simulink model "case 3"  (R2018a)
settings: Solver=VariableStepAuto  StartTime=0.0  StopTime=5  RelTol=1e-3
values from neighbouring files (symbols this model uses):
  cdcc = 0.00022    [matlab.mat]
  cf = 8e-05    [matlab.mat]
  iodmax = 12    [matlab.mat]
  iqdmax = -7.2    [matlab.mat]
  kiid = 0.5    [matlab.mat]
  kiiq = -5    [matlab.mat]
  kpid = 0.4    [matlab.mat]
  kpiq = -4    [matlab.mat]
  lf = 0.0075    [matlab.mat]
  ll = 1e-06    [matlab.mat]
  md = 0.001    [matlab.mat]
  nq = 0.002    [matlab.mat]
  p0 = 240    [matlab.mat]
  q0 = 60    [matlab.mat]
  rf = 0.0015    [matlab.mat]
  rl = 0.001    [matlab.mat]
  vdc = 200    [matlab.mat]
  wc = 0.000125663706144    [matlab.mat]
undefined symbols (not defined in the file or in its folder): DiscIntNeverNeededParam, gcbh, sps, sps_rtmsupport
libraries: neural x30, powerlib_meascontrol x27, powerlib x17, spsVIMeasurementModel x6, simulink x4, spsMeanValueModel x2
(part 1 of 2)
settings Model: Creator=Febin  LastModifiedBy=febin

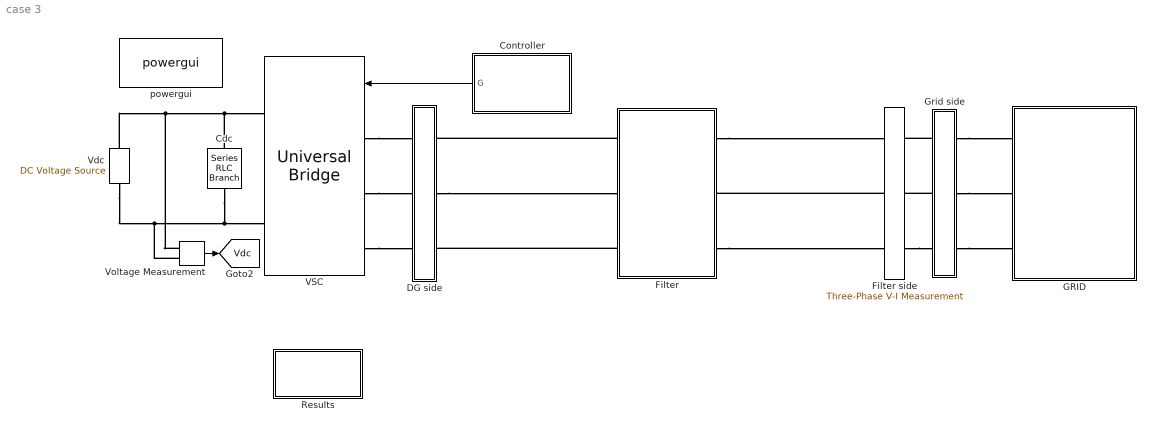
== system case 3 ==
  Cdc : powerlib/Elements/Series RLC Branch  LConnTagsString=__new0  RConnTagsString=__new0  BranchType=RC  Resistance=0.0001  Inductance=1e-3  SetiL0=off  InitialCurrent=0  Capacitance=cdcc  Setx0=off  InitialVoltage=0  Measurements=None
  Controller : Subsystem
  DG side : Subsystem  DialogController=POWERSYS.PowerSysDialog  LoadFcn=|  StartFcn=sps_rtmsupport('StartFcn',gcbh);  StopFcn=sps_rtmsupport('StopFcn',gcbh);  mask(Three-Phase VI Measurement){VoltageMeasurement=phase-to-ground, SetLabelV=on, LabelV=vabc, Vpu=off, VpuLL=off, CurrentMeasurement=yes, SetLabelI=on, LabelI=iabc, Ipu=off, Pbase=100e6, Vbase=500e3, OutputType=Complex, PhasorSimulation=off, PSBequivalent=0}
      | if ~strcmp(get_param(bdroot,'BlockDiagramType'),'library')
      |     set_param([gcb,'/Model'],'LinkStatus','restore');
      | end
      | sps_rtmsupport('LoadFcn',gcbh);
      mask prompts: VoltageMeasurement "Voltage measurement"; SetLabelV "Use a label"; LabelV "Signal label  (use a From block to collect this signal)"; Vpu "Voltages in pu,  based on peak value of nominal phase-to-ground voltage"; VpuLL "Voltages in pu,  based on peak value of nominal phase-to-phase  voltage"; CurrentMeasurement "Current measurement"; SetLabelI "Use a label"; LabelI "Signal label  (use a From block to collect this signal)"; Ipu "Currents in pu"; Pbase "Base power ( VA 3 phase)"; Vbase "Nominal voltage used for pu measurement (Vrms phase-phase) :"; OutputType "Output signals in:"; PhasorSimulation "Phasor simulation (internal use)"; PSBequivalent "Equivalent circuit (internal use)"
      mask help:
      | Ideal three-phase voltage and current measurements.
      |
      | The block can output the voltages and currents in per unit values or in volts and amperes.
      mask init:
      | block = gcb;
      | Kv=1;
      | Ki=1;
      | [Kv,Ki] = powericon('ThreePhaseVIMeasurementParam',block,Vpu,VpuLL,Ipu,Vbase,Pbase,PhasorSimulation,OutputType);
      | powericon('ThreePhaseVIMeasurementCback',block);
      | power_initmask();
      settings: CopyFcn=sps_rtmsupport('CopyFcn',gcbh); powericon('ThreePhaseVIMeasurementCopy',gcb)  DeleteFcn=sps_rtmsupport('DeleteFcn',gcbh);  UndoDeleteFcn=sps_rtmsupport('UndoDeleteFcn',gcbh);  ModelCloseFcn=sps_rtmsupport('ModelCloseFcn',gcbh);  PostSaveFcn=sps_rtmsupport('PostSaveFcn',gcbh);  NameChangeFcn=sps_rtmsupport('NameChangeFcn',gcbh);  PreCopyFcn=sps_rtmsupport('PreCopyFcn',gcbh);  OpenFcn=sps_rtmsupport('OpenFcn',gcbh, [1 2 4 5 6 7 9 -12 13]);  CloseFcn=sps_rtmsupport('CloseFcn',gcbh);  PreDeleteFcn=sps_rtmsupport('PreDeleteFcn',gcbh);
      settings: PreSaveFcn=|
      | sps_rtmsupport('PreSaveFcn',gcbh);
      | if ~strcmp(get_param(bdroot(gcbh),'BlockDiagramType'),'library')
      |     set_param(gcb,'LinkStatus','restore')
      | end
      mask Help: helpview(psbhelp)
      mask TypeOptions VoltageMeasurement: no | phase-to-ground | phase-to-phase
      mask Callback VoltageMeasurement: powericon('ThreePhaseVIMeasurementCback',gcb,'Vselector');
      mask Callback SetLabelV: powericon('ThreePhaseVIMeasurementCback',gcb,'');
      mask Callback Vpu: powericon('ThreePhaseVIMeasurementCback',gcb,'Vpu');
      mask Callback VpuLL: powericon('ThreePhaseVIMeasurementCback',gcb,'VpuLL');
      mask TypeOptions CurrentMeasurement: no | yes
      mask Callback CurrentMeasurement: powericon('ThreePhaseVIMeasurementCback',gcb,'');
      mask Callback SetLabelI: powericon('ThreePhaseVIMeasurementCback',gcb,'');
      mask Callback LabelI: powericon('ThreePhaseVIMeasurementCback',gcb,'');
      mask Callback Ipu: powericon('ThreePhaseVIMeasurementCback',gcb,'');
      mask TypeOptions OutputType: Complex | Real-Imag | Magnitude-Angle | Magnitude
  Filter : Subsystem
  Filter side : powerlib/Measurements/Three-Phase V-I Measurement  VoltageMeasurement=phase-to-ground  SetLabelV=on  LabelV=v0abc  Vpu=off  VpuLL=off  CurrentMeasurement=yes  SetLabelI=on  LabelI=i0abc  Ipu=off  Pbase=100e6  Vbase=500e3  OutputType=Complex  PhasorSimulation=off  PSBequivalent=0
  GRID : Subsystem
  Grid side : Subsystem  DialogController=POWERSYS.PowerSysDialog  LoadFcn=|  StartFcn=sps_rtmsupport('StartFcn',gcbh);  StopFcn=sps_rtmsupport('StopFcn',gcbh);  mask(Three-Phase VI Measurement){VoltageMeasurement=phase-to-ground, SetLabelV=on, LabelV=vgabc, Vpu=off, VpuLL=off, CurrentMeasurement=yes, SetLabelI=on, LabelI=igabc, Ipu=off, Pbase=100e6, Vbase=500e3, OutputType=Complex, PhasorSimulation=off, PSBequivalent=0}
      | if ~strcmp(get_param(bdroot,'BlockDiagramType'),'library')
      |     set_param([gcb,'/Model'],'LinkStatus','restore');
      | end
      | sps_rtmsupport('LoadFcn',gcbh);
      mask prompts: VoltageMeasurement "Voltage measurement"; SetLabelV "Use a label"; LabelV "Signal label  (use a From block to collect this signal)"; Vpu "Voltages in pu,  based on peak value of nominal phase-to-ground voltage"; VpuLL "Voltages in pu,  based on peak value of nominal phase-to-phase  voltage"; CurrentMeasurement "Current measurement"; SetLabelI "Use a label"; LabelI "Signal label  (use a From block to collect this signal)"; Ipu "Currents in pu"; Pbase "Base power ( VA 3 phase)"; Vbase "Nominal voltage used for pu measurement (Vrms phase-phase) :"; OutputType "Output signals in:"; PhasorSimulation "Phasor simulation (internal use)"; PSBequivalent "Equivalent circuit (internal use)"
      mask help:
      | Ideal three-phase voltage and current measurements.
      |
      | The block can output the voltages and currents in per unit values or in volts and amperes.
      mask init: same as case 3/DG side
      settings: CopyFcn=sps_rtmsupport('CopyFcn',gcbh); powericon('ThreePhaseVIMeasurementCopy',gcb)  DeleteFcn=sps_rtmsupport('DeleteFcn',gcbh);  UndoDeleteFcn=sps_rtmsupport('UndoDeleteFcn',gcbh);  ModelCloseFcn=sps_rtmsupport('ModelCloseFcn',gcbh);  PostSaveFcn=sps_rtmsupport('PostSaveFcn',gcbh);  NameChangeFcn=sps_rtmsupport('NameChangeFcn',gcbh);  PreCopyFcn=sps_rtmsupport('PreCopyFcn',gcbh);  OpenFcn=sps_rtmsupport('OpenFcn',gcbh, [1 2 4 5 6 7 9 -12 13]);  CloseFcn=sps_rtmsupport('CloseFcn',gcbh);  PreDeleteFcn=sps_rtmsupport('PreDeleteFcn',gcbh);
      settings: PreSaveFcn=|
      | sps_rtmsupport('PreSaveFcn',gcbh);
      | if ~strcmp(get_param(bdroot(gcbh),'BlockDiagramType'),'library')
      |     set_param(gcb,'LinkStatus','restore')
      | end
      mask Help: helpview(psbhelp)
      mask TypeOptions VoltageMeasurement: no | phase-to-ground | phase-to-phase
      mask Callback VoltageMeasurement: powericon('ThreePhaseVIMeasurementCback',gcb,'Vselector');
      mask Callback SetLabelV: powericon('ThreePhaseVIMeasurementCback',gcb,'');
      mask Callback Vpu: powericon('ThreePhaseVIMeasurementCback',gcb,'Vpu');
      mask Callback VpuLL: powericon('ThreePhaseVIMeasurementCback',gcb,'VpuLL');
      mask TypeOptions CurrentMeasurement: no | yes
      mask Callback CurrentMeasurement: powericon('ThreePhaseVIMeasurementCback',gcb,'');
      mask Callback SetLabelI: powericon('ThreePhaseVIMeasurementCback',gcb,'');
      mask Callback LabelI: powericon('ThreePhaseVIMeasurementCback',gcb,'');
      mask Callback Ipu: powericon('ThreePhaseVIMeasurementCback',gcb,'');
      mask TypeOptions OutputType: Complex | Real-Imag | Magnitude-Angle | Magnitude
  Results : Subsystem
  VSC : powerlib/Power Electronics/Universal Bridge  Arms=3  SnubberResistance=1e5  SnubberCapacitance=inf  Device=IGBT / Diodes  Ron=1e-3  Lon=0  ForwardVoltages="[  0  0  ]"  ForwardVoltage=0  GTOparameters=[ 10e-6 , 20e-6 ]  IGBTparameters=[ 1e-6 , 2e-6 ]  Measurements=None  Measurements_2=None  converterType=Rectifier
  Vdc : powerlib/Electrical Sources/DC Voltage Source  Amplitude=vdc  Measurements=None
  Voltage Measurement : powerlib/Measurements/Voltage Measurement  PhasorSimulation=off  OutputType=Complex  PSBequivalent=0
  powergui : powerlib/powergui  Priority=1  SimulationMode=Discrete  SampleTime=50e-6  frequency=60  Iterations=50  frequencyindice=0  Pbase=100e6  ErrMax=1e-4  UnitsV=kV  UnitsW=MW  buscounter=0  FunctionMessages=off  echomessages=off  EnableUseOfTLC=off  CurrentSourceSwitches=off  DisableSnubberDevices=off  DisableRonSwitches=off  DisableVfSwitches=off  DisplayEquations=off  SolverType=Tustin/Backward Euler (TBE)  Interpol=off  ExternalGateDelay=off  methode=off  Ts=100  x0status=blocks  SPID=off  SwTol=0  HookPort=off  RestoreLinks=warning  ResistiveCurrentMeasurement=off  Frange=[0:2:500]  Ylog=off  Xlog=on  ShowGrid=off  save=off  variable=ZData  structure=0  ZoomFFT=on  StartTime=0.0  cycles=1  DisplayStyle=1  fundamental=60  FreqAxis=off  MaxFrequency=1000  frequencyindicesteady=1  RmsSteady=1  display=off
  tag scope: Vdc=global
  wires:
  Controller/1(G) -> VSC/1
  Voltage Measurement/1 -> [Vdc]
  connections:
  Vdc/RConn1 -- Voltage Measurement/LConn1 -- Cdc/LConn1 -- VSC/RConn1
  Vdc/LConn1 -- Voltage Measurement/LConn2 -- Cdc/RConn1 -- VSC/RConn2
  VSC/LConn3 -- DG side/LConn3
  VSC/LConn2 -- DG side/LConn2
  VSC/LConn1 -- DG side/LConn1
  Grid side/RConn1 -- Filter side/LConn1
  Grid side/RConn2 -- Filter side/LConn2
  Filter side/LConn3 -- Grid side/RConn3
  Grid side/LConn1 -- GRID/RConn1
  Grid side/LConn2 -- GRID/RConn2
  Grid side/LConn3 -- GRID/RConn3
  Filter/LConn1 -- DG side/RConn1
  Filter/RConn1 -- Filter side/RConn1
  DG side/RConn2 -- Filter/LConn2
  Filter side/RConn2 -- Filter/RConn2
  Filter/LConn3 -- DG side/RConn3
  Filter/RConn3 -- Filter side/RConn3

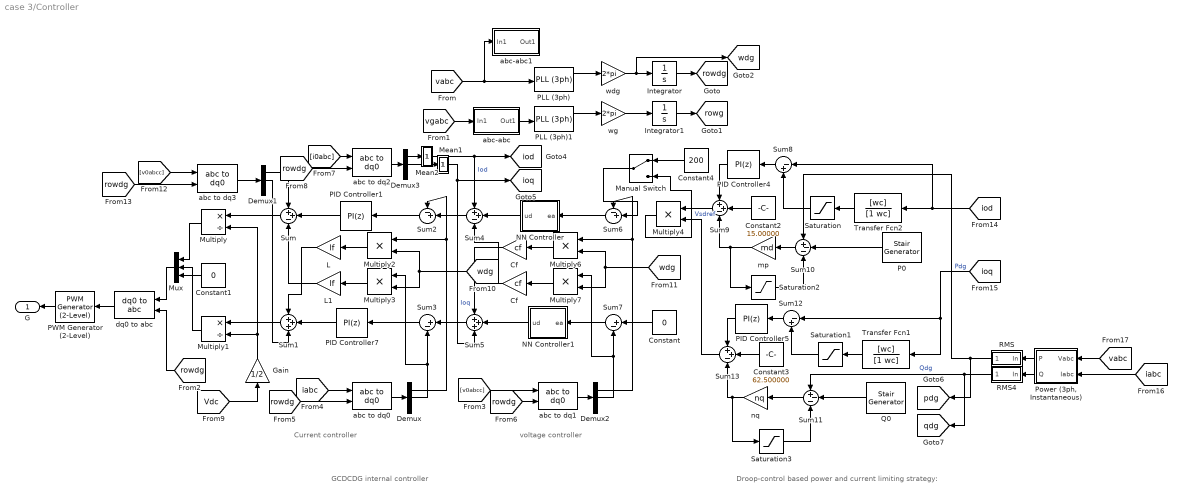
== system case 3/Controller ==
  note: voltage controller
  note: Current controller
  note: GCDCDG internal controller
  note: Droop-control based power and current limiting strategy:
  Cf : Gain  Gain=cf
  "Cf " : Gain  Gain=cf
  Constant : Constant  Value=0
  Constant1 : Constant  Value=0
  Constant2 : Constant  Value=15.00000
  Constant3 : Constant  Value=62.500000
  Constant4 : Constant  Value=200
  Demux{,1..3} (4 alike) : Demux  Outputs=3
  Gain : Gain  Gain=1/2
  Integrator : Integrator
  Integrator1 : Integrator
  L : Gain  Gain=lf
  L1 : Gain  Gain=lf
  Manual Switch : ManualSwitch
  Mean1 : Subsystem  DialogController=POWERSYS.PowerSysDialog  LoadFcn=sps_rtmsupport('LoadFcn', gcbh);  StartFcn=sps_rtmsupport('StartFcn', gcbh);  StopFcn=sps_rtmsupport('StopFcn', gcbh);  mask(Mean){Freq=50, Vinit=0, Ts=50e-6}
      mask prompts: Freq "Fundamental frequency (Hz):"; Vinit "Initial input (DC component):"; Ts "Sample time:"
      mask help: Compute the mean value of the input signal over a running window of one cycle of the specified fundamental frequency. For the first cycle of simulation, the output is held constant to the specified initial input value.
      mask init:
      | block=gcb;
      | [WantBlockChoice,Ts,sps] = powericon('MeanInit',block,Freq,Vinit,Ts);
      | powericon('SetInternalModels','set',block,WantBlockChoice);
      settings: CopyFcn=sps_rtmsupport('CopyFcn', gcbh);  DeleteFcn=sps_rtmsupport('DeleteFcn', gcbh);  UndoDeleteFcn=sps_rtmsupport('UndoDeleteFcn', gcbh);  ModelCloseFcn=sps_rtmsupport('ModelCloseFcn', gcbh);  PreSaveFcn=sps_rtmsupport('PreSaveFcn', gcbh);  PostSaveFcn=sps_rtmsupport('PostSaveFcn', gcbh);  NameChangeFcn=sps_rtmsupport('NameChangeFcn', gcbh);  PreCopyFcn=sps_rtmsupport('PreCopyFcn', gcbh);  OpenFcn=sps_rtmsupport('OpenFcn', gcbh, []);  CloseFcn=sps_rtmsupport('CloseFcn', gcbh);  PreDeleteFcn=sps_rtmsupport('PreDeleteFcn', gcbh);
      mask Help: helpview(psbhelp);
      mask Display:
      | plot(0,0, 1,1)
      | plot([0.8 1], [0.75 0.75])
      | plot([0.85 .95], [0.35 0.65],[0.85 .95], [0.65 0.35])
  Mean2 : Subsystem  DialogController=POWERSYS.PowerSysDialog  LoadFcn=sps_rtmsupport('LoadFcn', gcbh);  StartFcn=sps_rtmsupport('StartFcn', gcbh);  StopFcn=sps_rtmsupport('StopFcn', gcbh);  mask(Mean){Freq=50, Vinit=0, Ts=50e-6}
      mask prompts: Freq "Fundamental frequency (Hz):"; Vinit "Initial input (DC component):"; Ts "Sample time:"
      mask help: Compute the mean value of the input signal over a running window of one cycle of the specified fundamental frequency. For the first cycle of simulation, the output is held constant to the specified initial input value.
      mask init:
      | block=gcb;
      | [WantBlockChoice,Ts,sps] = powericon('MeanInit',block,Freq,Vinit,Ts);
      | powericon('SetInternalModels','set',block,WantBlockChoice);
      settings: CopyFcn=sps_rtmsupport('CopyFcn', gcbh);  DeleteFcn=sps_rtmsupport('DeleteFcn', gcbh);  UndoDeleteFcn=sps_rtmsupport('UndoDeleteFcn', gcbh);  ModelCloseFcn=sps_rtmsupport('ModelCloseFcn', gcbh);  PreSaveFcn=sps_rtmsupport('PreSaveFcn', gcbh);  PostSaveFcn=sps_rtmsupport('PostSaveFcn', gcbh);  NameChangeFcn=sps_rtmsupport('NameChangeFcn', gcbh);  PreCopyFcn=sps_rtmsupport('PreCopyFcn', gcbh);  OpenFcn=sps_rtmsupport('OpenFcn', gcbh, []);  CloseFcn=sps_rtmsupport('CloseFcn', gcbh);  PreDeleteFcn=sps_rtmsupport('PreDeleteFcn', gcbh);
      mask Help: helpview(psbhelp);
      mask Display:
      | plot(0,0, 1,1)
      | plot([0.8 1], [0.75 0.75])
      | plot([0.85 .95], [0.35 0.65],[0.85 .95], [0.65 0.35])
  Multiply : Product  Inputs=*/
  Multiply1 : Product  Inputs=*/
  Multiply{2..4,6..7} (5 alike) : Product
  Mux : Mux  Inputs=3
  NN Controller : Subsystem
  NN Controller1 : Subsystem
  P0 : powerlib_meascontrol/Pulse & Signal Generators/Stair Generator  t=[0 2 5]  e=[1 1 1]*p0  Ts=50e-6
      settings: SourceProductName=Simscape Power Systems
  PID Controller1 : simulink/Continuous/PID Controller  Controller=PI  TimeDomain=Discrete-time  SampleTime=-1  IntegratorMethod=Forward Euler  FilterMethod=Forward Euler  Form=Parallel  UseFilter=on  ControllerParametersSource=internal  P=0.2  I=0.01  D=0  N=100  InitialConditionSource=internal  InitialConditionForIntegrator=0  InitialConditionForFilter=0  ExternalReset=none  LimitOutput=off  UpperSaturationLimit=1  LowerSaturationLimit=-1  LinearizeAsGain=on  AntiWindupMode=none  Kb=1  TrackingMode=off  Kt=1  PParamMin=[]  PParamMax=[]  IParamMin=[]  IParamMax=[]  DParamMin=[]  DParamMax=[]  NParamMin=[]  NParamMax=[]  KbParamMin=[]  KbParamMax=[]  KtParamMin=[]  KtParamMax=[]  POutMin=[]  POutMax=[]  IOutMin=[]  IOutMax=[]  DOutMin=[]  DOutMax=[]  NOutMin=[]  NOutMax=[]  KbOutMin=[]  KbOutMax=[]  KtOutMin=[]  KtOutMax=[]  IntegratorOutMin=[]  IntegratorOutMax=[]  FilterOutMin=[]  FilterOutMax=[]  SumOutMin=[]  SumOutMax=[]  SumI1OutMin=[]  SumI1OutMax=[]  SumI2OutMin=[]  SumI2OutMax=[]  SumI3OutMin=[]  SumI3OutMax=[]  SumDOutMin=[]  SumDOutMax=[]  SaturationOutMin=[]  SaturationOutMax=[]  IntegratorContinuousStateAttributes=''  IntegratorStateMustResolveToSignalObject=off  IntegratorRTWStateStorageClass=Auto  FilterContinuousStateAttributes=''  FilterStateMustResolveToSignalObject=off  FilterRTWStateStorageClass=Auto  DifferentiatorICPrevScaledInput=0  DifferentiatorOutMin=[]  DifferentiatorOutMax=[]  FilterDiffOutCoefMin=[]  FilterDiffOutCoefMax=[]  SumDenOutMin=[]  SumDenOutMax=[]  SumNumOutMin=[]  SumNumOutMax=[]  ReciprocalOutMin=[]  ReciprocalOutMax=[]  DivideOutMin=[]  DivideOutMax=[]  TunerSelectOption=Transfer Function Based (PID Tuner App)
  PID Controller4 : simulink/Continuous/PID Controller  Controller=PI  TimeDomain=Discrete-time  SampleTime=-1  IntegratorMethod=Forward Euler  FilterMethod=Forward Euler  Form=Parallel  UseFilter=on  ControllerParametersSource=internal  P=kpid  I=kpiq  D=0  N=100  InitialConditionSource=internal  InitialConditionForIntegrator=0  InitialConditionForFilter=0  ExternalReset=none  LimitOutput=off  UpperSaturationLimit=inf  LowerSaturationLimit=-inf  LinearizeAsGain=on  AntiWindupMode=none  Kb=1  TrackingMode=off  Kt=1  PParamMin=[]  PParamMax=[]  IParamMin=[]  IParamMax=[]  DParamMin=[]  DParamMax=[]  NParamMin=[]  NParamMax=[]  KbParamMin=[]  KbParamMax=[]  KtParamMin=[]  KtParamMax=[]  POutMin=[]  POutMax=[]  IOutMin=[]  IOutMax=[]  DOutMin=[]  DOutMax=[]  NOutMin=[]  NOutMax=[]  KbOutMin=[]  KbOutMax=[]  KtOutMin=[]  KtOutMax=[]  IntegratorOutMin=[]  IntegratorOutMax=[]  FilterOutMin=[]  FilterOutMax=[]  SumOutMin=[]  SumOutMax=[]  SumI1OutMin=[]  SumI1OutMax=[]  SumI2OutMin=[]  SumI2OutMax=[]  SumI3OutMin=[]  SumI3OutMax=[]  SumDOutMin=[]  SumDOutMax=[]  SaturationOutMin=[]  SaturationOutMax=[]  IntegratorContinuousStateAttributes=''  IntegratorStateMustResolveToSignalObject=off  IntegratorRTWStateStorageClass=Auto  FilterContinuousStateAttributes=''  FilterStateMustResolveToSignalObject=off  FilterRTWStateStorageClass=Auto  DifferentiatorICPrevScaledInput=0  DifferentiatorOutMin=[]  DifferentiatorOutMax=[]  FilterDiffOutCoefMin=[]  FilterDiffOutCoefMax=[]  SumDenOutMin=[]  SumDenOutMax=[]  SumNumOutMin=[]  SumNumOutMax=[]  ReciprocalOutMin=[]  ReciprocalOutMax=[]  DivideOutMin=[]  DivideOutMax=[]  TunerSelectOption=Transfer Function Based (PID Tuner App)
  PID Controller5 : simulink/Continuous/PID Controller  Controller=PI  TimeDomain=Discrete-time  SampleTime=-1  IntegratorMethod=Forward Euler  FilterMethod=Forward Euler  Form=Parallel  UseFilter=on  ControllerParametersSource=internal  P=kiid  I=kiiq  D=0  N=100  InitialConditionSource=internal  InitialConditionForIntegrator=0  InitialConditionForFilter=0  ExternalReset=none  LimitOutput=off  UpperSaturationLimit=inf  LowerSaturationLimit=-inf  LinearizeAsGain=on  AntiWindupMode=none  Kb=1  TrackingMode=off  Kt=1  PParamMin=[]  PParamMax=[]  IParamMin=[]  IParamMax=[]  DParamMin=[]  DParamMax=[]  NParamMin=[]  NParamMax=[]  KbParamMin=[]  KbParamMax=[]  KtParamMin=[]  KtParamMax=[]  POutMin=[]  POutMax=[]  IOutMin=[]  IOutMax=[]  DOutMin=[]  DOutMax=[]  NOutMin=[]  NOutMax=[]  KbOutMin=[]  KbOutMax=[]  KtOutMin=[]  KtOutMax=[]  IntegratorOutMin=[]  IntegratorOutMax=[]  FilterOutMin=[]  FilterOutMax=[]  SumOutMin=[]  SumOutMax=[]  SumI1OutMin=[]  SumI1OutMax=[]  SumI2OutMin=[]  SumI2OutMax=[]  SumI3OutMin=[]  SumI3OutMax=[]  SumDOutMin=[]  SumDOutMax=[]  SaturationOutMin=[]  SaturationOutMax=[]  IntegratorContinuousStateAttributes=''  IntegratorStateMustResolveToSignalObject=off  IntegratorRTWStateStorageClass=Auto  FilterContinuousStateAttributes=''  FilterStateMustResolveToSignalObject=off  FilterRTWStateStorageClass=Auto  DifferentiatorICPrevScaledInput=0  DifferentiatorOutMin=[]  DifferentiatorOutMax=[]  FilterDiffOutCoefMin=[]  FilterDiffOutCoefMax=[]  SumDenOutMin=[]  SumDenOutMax=[]  SumNumOutMin=[]  SumNumOutMax=[]  ReciprocalOutMin=[]  ReciprocalOutMax=[]  DivideOutMin=[]  DivideOutMax=[]  TunerSelectOption=Transfer Function Based (PID Tuner App)
  PID Controller7 : simulink/Continuous/PID Controller  Controller=PI  TimeDomain=Discrete-time  SampleTime=-1  IntegratorMethod=Forward Euler  FilterMethod=Forward Euler  Form=Parallel  UseFilter=on  ControllerParametersSource=internal  P=0.2  I=0.01  D=0  N=100  InitialConditionSource=internal  InitialConditionForIntegrator=0  InitialConditionForFilter=0  ExternalReset=none  LimitOutput=off  UpperSaturationLimit=1  LowerSaturationLimit=-1  LinearizeAsGain=on  AntiWindupMode=none  Kb=1  TrackingMode=off  Kt=1  PParamMin=[]  PParamMax=[]  IParamMin=[]  IParamMax=[]  DParamMin=[]  DParamMax=[]  NParamMin=[]  NParamMax=[]  KbParamMin=[]  KbParamMax=[]  KtParamMin=[]  KtParamMax=[]  POutMin=[]  POutMax=[]  IOutMin=[]  IOutMax=[]  DOutMin=[]  DOutMax=[]  NOutMin=[]  NOutMax=[]  KbOutMin=[]  KbOutMax=[]  KtOutMin=[]  KtOutMax=[]  IntegratorOutMin=[]  IntegratorOutMax=[]  FilterOutMin=[]  FilterOutMax=[]  SumOutMin=[]  SumOutMax=[]  SumI1OutMin=[]  SumI1OutMax=[]  SumI2OutMin=[]  SumI2OutMax=[]  SumI3OutMin=[]  SumI3OutMax=[]  SumDOutMin=[]  SumDOutMax=[]  SaturationOutMin=[]  SaturationOutMax=[]  IntegratorContinuousStateAttributes=''  IntegratorStateMustResolveToSignalObject=off  IntegratorRTWStateStorageClass=Auto  FilterContinuousStateAttributes=''  FilterStateMustResolveToSignalObject=off  FilterRTWStateStorageClass=Auto  DifferentiatorICPrevScaledInput=0  DifferentiatorOutMin=[]  DifferentiatorOutMax=[]  FilterDiffOutCoefMin=[]  FilterDiffOutCoefMax=[]  SumDenOutMin=[]  SumDenOutMax=[]  SumNumOutMin=[]  SumNumOutMax=[]  ReciprocalOutMin=[]  ReciprocalOutMax=[]  DivideOutMin=[]  DivideOutMax=[]  TunerSelectOption=Transfer Function Based (PID Tuner App)
  PLL (3ph) : powerlib_meascontrol/PLL/PLL (3ph)  Fmin=45  Par_Init=[0, 50]  ParK=[180, 3200, 1]  TcD=1e-4  MaxRateChangeFreq=12  FilterCutOffFreq=25  Ts=50e-6  AGC=on
  PLL (3ph)1 : powerlib_meascontrol/PLL/PLL (3ph)  Fmin=45  Par_Init=[0, 50]  ParK=[180, 3200, 1]  TcD=1e-4  MaxRateChangeFreq=12  FilterCutOffFreq=25  Ts=50e-6  AGC=on
  PWM Generator (2-Level) : powerlib_meascontrol/Pulse & Signal Generators/PWM Generator (2-Level)  ModulatorType=Three-phase bridge (6 pulses)  ModulatorMode=Unsynchronized  Fc=2000  Pc=90  nF=27  MinMax="[ -1  1 ]"  SamplingTechnique=Natural  ModulatingSignals=off  m=0.8  Freq=60  Phase=0  Ts=50e-6  ShowCarrierOutport=off
      settings: SourceProductName=Simscape Power Systems
  "Power (3ph, Instantaneous)" : Subsystem  DialogController=POWERSYS.PowerSysDialog  LoadFcn=sps_rtmsupport('LoadFcn', gcbh);  StartFcn=sps_rtmsupport('StartFcn', gcbh);  StopFcn=sps_rtmsupport('StopFcn', gcbh);  mask(Power (3ph, Instantaneous)){}
      mask help:
      | Compute the three-phase instantaneous active and reactive powers associated with a periodic set of three-phase voltages and currents.
      |
      | Instantaneous reactive power is accurate only for balanced and harmonic-free three-phase voltages and currents.
      |
      | Current flowing into an RL circuit will produce positive active and reactive power.
      settings: CopyFcn=sps_rtmsupport('CopyFcn', gcbh);  DeleteFcn=sps_rtmsupport('DeleteFcn', gcbh);  UndoDeleteFcn=sps_rtmsupport('UndoDeleteFcn', gcbh);  ModelCloseFcn=sps_rtmsupport('ModelCloseFcn', gcbh);  PreSaveFcn=sps_rtmsupport('PreSaveFcn', gcbh);  PostSaveFcn=sps_rtmsupport('PostSaveFcn', gcbh);  NameChangeFcn=sps_rtmsupport('NameChangeFcn', gcbh);  PreCopyFcn=sps_rtmsupport('PreCopyFcn', gcbh);  OpenFcn=sps_rtmsupport('OpenFcn', gcbh, []);  CloseFcn=sps_rtmsupport('CloseFcn', gcbh);  PreDeleteFcn=sps_rtmsupport('PreDeleteFcn', gcbh);
      mask Help: helpview(psbhelp);
  Q0 : powerlib_meascontrol/Pulse & Signal Generators/Stair Generator  t=[0 2 5]  e=[1 1 1]*q0  Ts=0
      settings: SourceProductName=Simscape Power Systems
  RMS : Subsystem  DialogController=POWERSYS.PowerSysDialog  LoadFcn=sps_rtmsupport('LoadFcn', gcbh);  StartFcn=sps_rtmsupport('StartFcn', gcbh);  StopFcn=sps_rtmsupport('StopFcn', gcbh);  mask(RMS){TrueRMS=on, Freq=50, RMSInit=0, Ts=50e-6}
      mask prompts: TrueRMS "True RMS value"; Freq "Fundamental frequency (Hz):"; RMSInit "Initial RMS value:"; Ts "Sample time:"
      mask help:
      | Measure the true root mean square (RMS) value of the input signal at the specified fundamental frequency.
      |
      | When True RMS value parameter is unchecked, the block outputs the RMS value of the fundamental component of the input signal.
      mask init:
      | [sps] = powericon('RMSInit',gcb,Freq,RMSInit,TrueRMS,Ts);
      settings: CopyFcn=sps_rtmsupport('CopyFcn', gcbh);  DeleteFcn=sps_rtmsupport('DeleteFcn', gcbh);  UndoDeleteFcn=sps_rtmsupport('UndoDeleteFcn', gcbh);  ModelCloseFcn=sps_rtmsupport('ModelCloseFcn', gcbh);  PreSaveFcn=sps_rtmsupport('PreSaveFcn', gcbh);  PostSaveFcn=sps_rtmsupport('PostSaveFcn', gcbh);  NameChangeFcn=sps_rtmsupport('NameChangeFcn', gcbh);  PreCopyFcn=sps_rtmsupport('PreCopyFcn', gcbh);  OpenFcn=sps_rtmsupport('OpenFcn', gcbh, [1]);  CloseFcn=sps_rtmsupport('CloseFcn', gcbh);  PreDeleteFcn=sps_rtmsupport('PreDeleteFcn', gcbh);
      mask Help: helpview(psbhelp);
      mask Display: color('blue');disp('RMS')
  RMS4 : Subsystem  DialogController=POWERSYS.PowerSysDialog  LoadFcn=sps_rtmsupport('LoadFcn', gcbh);  StartFcn=sps_rtmsupport('StartFcn', gcbh);  StopFcn=sps_rtmsupport('StopFcn', gcbh);  mask(RMS){TrueRMS=on, Freq=50, RMSInit=0, Ts=50e-6}
      mask prompts: TrueRMS "True RMS value"; Freq "Fundamental frequency (Hz):"; RMSInit "Initial RMS value:"; Ts "Sample time:"
      mask help:
      | Measure the true root mean square (RMS) value of the input signal at the specified fundamental frequency.
      |
      | When True RMS value parameter is unchecked, the block outputs the RMS value of the fundamental component of the input signal.
      mask init:
      | [sps] = powericon('RMSInit',gcb,Freq,RMSInit,TrueRMS,Ts);
      settings: CopyFcn=sps_rtmsupport('CopyFcn', gcbh);  DeleteFcn=sps_rtmsupport('DeleteFcn', gcbh);  UndoDeleteFcn=sps_rtmsupport('UndoDeleteFcn', gcbh);  ModelCloseFcn=sps_rtmsupport('ModelCloseFcn', gcbh);  PreSaveFcn=sps_rtmsupport('PreSaveFcn', gcbh);  PostSaveFcn=sps_rtmsupport('PostSaveFcn', gcbh);  NameChangeFcn=sps_rtmsupport('NameChangeFcn', gcbh);  PreCopyFcn=sps_rtmsupport('PreCopyFcn', gcbh);  OpenFcn=sps_rtmsupport('OpenFcn', gcbh, [1]);  CloseFcn=sps_rtmsupport('CloseFcn', gcbh);  PreDeleteFcn=sps_rtmsupport('PreDeleteFcn', gcbh);
      mask Help: helpview(psbhelp);
      mask Display: color('blue');disp('RMS')
  Saturation : Saturate  UpperLimit=iodmax  LowerLimit=0
  Saturation1 : Saturate  UpperLimit=0  LowerLimit=iqdmax
  Saturation2 : Saturate  UpperLimit=p0  LowerLimit=0
  Saturation3 : Saturate  UpperLimit=q0  LowerLimit=0
  Sum{,4,9,13} (4 alike) : Sum  Inputs=++-
  Sum1 : Sum  Inputs=+++
  Sum10 : Sum  Inputs=+--
  Sum11 : Sum  Inputs=+--
  Sum12 : Sum  Inputs=|-+
  Sum2 : Sum  Inputs=-+|
  Sum3 : Sum  Inputs=|+-
  Sum5 : Sum  Inputs=+++
  Sum6 : Sum  Inputs=-+|
  Sum7 : Sum  Inputs=|+-
  Sum8 : Sum  Inputs=|-+
  Transfer Fcn1 : TransferFcn  Numerator=[wc]  Denominator=[1 wc]
  Transfer Fcn2 : TransferFcn  Numerator=[wc]  Denominator=[1 wc]
  abc to dq{0..3} (4 alike) : powerlib_meascontrol/Transformations/abc to dq0  Alignment=90 degrees behind phase A axis
  abc-abc : Subsystem
  abc-abc1 : Subsystem
  dq0 to abc : powerlib_meascontrol/Transformations/dq0 to abc  Alignment=90 degrees behind phase A axis
  mp : Gain  Gain=md
  nq : Gain  Gain=nq
  wdg : Gain  Gain=2*pi
  wg : Gain  Gain=2*pi
  G : Outport
  tag scope: iod=global, ioq=global, pdg=global, qdg=global, rowdg=global, rowg=global, wdg=global
  wires:
  PWM Generator (2-Level)/1 -> G/1
  wg/1 -> Integrator1/1
  [iabc] -> abc to dq0/1
  dq0 to abc/1 -> PWM Generator (2-Level)/1
  [i0abc] -> abc to dq2/1
  [vgabc] -> abc-abc/1(In1)
  [rowdg] -> abc to dq2/2
  [rowdg] -> abc to dq0/2
  Integrator/1 -> [rowdg]
  Integrator1/1 -> [rowg]
  Mux/1 -> dq0 to abc/1
  [Vdc] -> Gain/1
  Gain/1 -> Multiply/2, Multiply1/2
  Sum/1 -> Multiply/1
  Sum1/1 -> Multiply1/1
  Sum2/1 -> PID Controller1/1
  PID Controller1/1 -> Sum/2
  Multiply/1 -> Mux/1
  Multiply1/1 -> Mux/2
  Multiply2/1 -> L/1
  Multiply3/1 -> L1/1
  abc to dq0/1 -> Demux/1
  abc to dq3/1 -> Demux1/1
  Demux1/1 -> Sum/1
  Demux1/2 -> Sum1/3
  Demux/1 -> Multiply2/1, Sum2/1
  Demux/2 -> Multiply3/1, Sum3/2
  [wdg] -> Multiply2/2, Multiply3/2
  abc to dq1/1 -> Demux2/1
  Demux2/2 -> Multiply7/1, Sum7/2
  Multiply7/1 -> "Cf "/1
  Multiply6/1 -> Cf/1
  Sum6/1 -> NN Controller/1(ea)
  Demux2/1 -> Multiply6/1, Sum6/1
  [wdg] -> Multiply7/2, Multiply6/2
  Sum4/1 -> Sum2/2
  Sum5/1 -> Sum3/1
  abc to dq2/1 -> Demux3/1
  Constant/1 -> Sum7/1
  Constant1/1 -> Mux/3
  [v0abcc] -> abc to dq1/1
  [rowdg] -> abc to dq1/2
  [rowdg] -> abc to dq3/2
  [v0abcc] -> abc to dq3/1
  [iod] -> Transfer Fcn2/1, Sum8/1
  Saturation/1 -> Sum8/2
  Transfer Fcn2/1 -> Saturation/1
  Sum8/1 -> PID Controller4/1
  mp/1 -> Saturation2/1, Sum9/3
  [vabc] -> "Power (3ph, Instantaneous)"/1(Vabc)
  [iabc] -> "Power (3ph, Instantaneous)"/2(Iabc)
  P0/1 -> Sum10/2
  Sum10/1 -> mp/1
  nq/1 -> Saturation3/1, Sum13/3
  Q0/1 -> Sum11/2
  Sum11/1 -> nq/1
  Sum12/1 -> PID Controller5/1
  Transfer Fcn1/1 -> Saturation1/1
  Saturation1/1 -> Sum12/2
  [ioq] -> Sum12/1, Transfer Fcn1/1
  Sum9/1 -> Multiply4/1
  Sum13/1 -> Multiply4/2
  Constant2/1 -> Sum9/2
  Constant3/1 -> Sum13/2
  PID Controller4/1 -> Sum9/1
  PID Controller5/1 -> Sum13/1
  Saturation2/1 -> Sum10/3
  Saturation3/1 -> Sum11/3
  abc-abc/1(Out1) -> PLL (3ph)1/1
  PLL (3ph)1/1 -> wg/1
  Constant4/1 -> Manual Switch/1
  Multiply4/1 -> Manual Switch/2  "Vsdref"
  Manual Switch/1 -> Sum6/2
  Sum7/1 -> NN Controller1/1(ea)
  NN Controller/1(ud) -> Sum4/2
  NN Controller1/1(ud) -> Sum5/2
  Sum3/1 -> PID Controller7/1
  "Cf "/1 -> Sum4/3
  Cf/1 -> Sum5/1
  L1/1 -> Sum/3
  L/1 -> Sum1/1
  PID Controller7/1 -> Sum1/2
  PLL (3ph)/1 -> wdg/1
  [rowdg] -> dq0 to abc/2
  wdg/1 -> [wdg], Integrator/1
  [vabc] -> abc-abc1/1(In1), PLL (3ph)/1
  Demux3/2 -> Mean1/1(In)
  Demux3/1 -> Mean2/1(In)
  Mean2/1(Mean) -> Sum4/1, [iod]  "Iod"
  Mean1/1(Mean) -> [ioq], Sum5/3  "Ioq"
  "Power (3ph, Instantaneous)"/1(P) -> RMS/1(In)
  "Power (3ph, Instantaneous)"/2(Q) -> RMS4/1(In)
  RMS/1(RMS) -> [pdg], Sum10/1  "Pdg"
  RMS4/1(RMS) -> [qdg], Sum11/1  "Qdg"

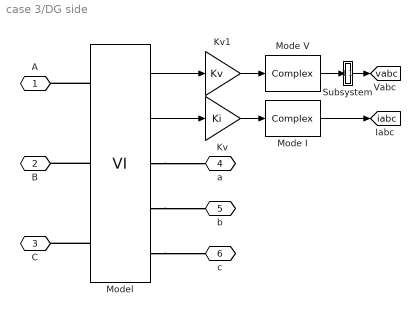
== system case 3/DG side ==
  Kv : Gain  Gain=Ki  SaturateOnIntegerOverflow=on  OutDataTypeStr=Inherit: Same as input  ParamDataTypeStr=Inherit: Same as input
  Kv1 : Gain  Gain=Kv  SaturateOnIntegerOverflow=on  OutDataTypeStr=Inherit: Same as input  ParamDataTypeStr=Inherit: Same as input
  Mode I : spsVIMeasurementModel/Complex
  Mode V : spsVIMeasurementModel/Complex
  Model : spsVIMeasurementModel/VI  SystemSampleTime=-1
  Subsystem : Subsystem
  A : PMIOPort  Side=Left
  B : PMIOPort  Port=2  Side=Left
  C : PMIOPort  Port=3  Side=Left
  a : PMIOPort  Port=4  Side=Right
  b : PMIOPort  Port=5  Side=Right
  c : PMIOPort  Port=6  Side=Right
  tag scope: iabc=global, vabc=global
  wires:
  Model/2 -> Kv/1
  Model/1 -> Kv1/1
  Kv/1 -> Mode I/1
  Kv1/1 -> Mode V/1
  Mode V/1 -> Subsystem/1(In1)
  Subsystem/1(Out2) -> [vabc]
  Mode I/1 -> [iabc]
  connections:
  Model/RConn3 -- c/RConn1
  Model/RConn1 -- a/RConn1
  Model/RConn2 -- b/RConn1
  Model/LConn3 -- C/RConn1
  Model/LConn1 -- A/RConn1
  Model/LConn2 -- B/RConn1

== system case 3/Filter ==
  Cf : powerlib/Elements/Three-Phase Series RLC Branch  LConnTagsString=A|B|C  RConnTagsString=A|B|C  BranchType=C  Resistance=0.00001  Inductance=1e-3  Capacitance=cf  Measurements=None
  "Lf " : powerlib/Elements/Three-Phase Series RLC Branch  LConnTagsString=A|B|C  RConnTagsString=A|B|C  BranchType=L  Resistance=rf  Inductance=lf  Capacitance=1e-6  Measurements=None
  Three-Phase V-I Measurement3 : powerlib/Measurements/Three-Phase V-I Measurement  VoltageMeasurement=phase-to-ground  SetLabelV=on  LabelV=v0abcc  Vpu=off  VpuLL=off  CurrentMeasurement=yes  SetLabelI=on  LabelI=i0abcc  Ipu=off  Pbase=100e6  Vbase=500e3  OutputType=Complex  PhasorSimulation=off  PSBequivalent=0
  a : PMIOPort  Side=Left
  A : PMIOPort  Port=2  Side=Right
  b : PMIOPort  Port=3  Side=Left
  B : PMIOPort  Port=4  Side=Right
  c : PMIOPort  Port=5  Side=Left
  C : PMIOPort  Port=6  Side=Right
  connections:
  Cf/LConn3 -- Three-Phase V-I Measurement3/RConn1
  "Lf "/RConn1 -- A/RConn1 -- Three-Phase V-I Measurement3/LConn3
  Cf/RConn1 -- Cf/RConn3 -- Cf/RConn2
  "Lf "/RConn3 -- C/RConn1 -- Three-Phase V-I Measurement3/LConn1
  Cf/LConn1 -- Three-Phase V-I Measurement3/RConn3
  b/RConn1 -- "Lf "/LConn2
  Cf/LConn2 -- Three-Phase V-I Measurement3/RConn2
  Three-Phase V-I Measurement3/LConn2 -- B/RConn1 -- "Lf "/RConn2
  "Lf "/LConn3 -- c/RConn1
  "Lf "/LConn1 -- a/RConn1

== system case 3/GRID ==
  Ground : powerlib/Elements/Ground  LConnTagsString=a
  Ground1 : powerlib/Elements/Ground  LConnTagsString=a
  LC : powerlib/Elements/Three-Phase Series RLC Branch  LConnTagsString=A|B|C  RConnTagsString=A|B|C  BranchType=RL  Resistance=rl  Inductance=ll  Capacitance=1e-6  Measurements=None
  LC1 : powerlib/Elements/Three-Phase Series RLC Branch  LConnTagsString=A|B|C  RConnTagsString=A|B|C  BranchType=RL  Resistance=rl  Inductance=ll  Capacitance=1e-6  Measurements=None
  Three-Phase Programmable Voltage Source : powerlib/Electrical Sources/Three-Phase Programmable Voltage Source  PositiveSequence="[200  0 50]"  VariationEntity=None  VariationType=Table of time-amplitude pairs  VariationTypeAlt=Step  VariationStep=0.5  VariationRate=10  VariationMagnitude=0.3  VariationFrequency=2  VariationTiming=[1 2]  VariationPhaseA=off  Amplitudes=[1 0.8 1.2 1.0]  TimeValues=[0 0.1 0.15 0.2]  HarmonicGeneration=off  HarmonicA=[3 0.2 -25 0]  HarmonicB=[2 0.15 35 2]  Timing="[0.05  3]"  BusType=swing  Pref=0  Qref=0  Qmin=-inf  Qmax=inf
  Three-Phase Programmable Voltage Source1 : powerlib/Electrical Sources/Three-Phase Programmable Voltage Source  PositiveSequence="[200*0.44  0 50]"  VariationEntity=None  VariationType=Table of time-amplitude pairs  VariationTypeAlt=Step  VariationStep=0.5  VariationRate=10  VariationMagnitude=0.3  VariationFrequency=2  VariationTiming=[1 2]  VariationPhaseA=off  Amplitudes=[1 0.8 1.2 1.0]  TimeValues=[0 0.1 0.15 0.2]  HarmonicGeneration=off  HarmonicA=[3 0.2 -25 0]  HarmonicB=[2 0.15 35 2]  Timing="[0.05  3]"  BusType=swing  Pref=0  Qref=0  Qmin=-inf  Qmax=inf
  Three-Phase Breaker : powerlib/Elements/Three-Phase Breaker  InitialState=open  SwitchA=on  SwitchB=on  SwitchC=on  SwitchTimes=[0 2]  External=off  BreakerResistance=0.01  SnubberResistance=1e6  SnubberCapacitance=inf  Measurements=None
  Three-Phase Breaker1 : powerlib/Elements/Three-Phase Breaker  InitialState=closed  SwitchA=on  SwitchB=on  SwitchC=on  SwitchTimes=[0 2]  External=off  BreakerResistance=0.01  SnubberResistance=1e6  SnubberCapacitance=inf  Measurements=None
  A : PMIOPort  Side=Right
  B : PMIOPort  Port=2  Side=Right
  C : PMIOPort  Port=3  Side=Right
  connections:
  Three-Phase Programmable Voltage Source/LConn1 -- Ground/LConn1
  LC/RConn1 -- Three-Phase Programmable Voltage Source/RConn1
  Three-Phase Programmable Voltage Source/RConn2 -- LC/RConn2
  LC/RConn3 -- Three-Phase Programmable Voltage Source/RConn3
  LC1/RConn3 -- Three-Phase Programmable Voltage Source1/RConn3
  Three-Phase Programmable Voltage Source1/RConn2 -- LC1/RConn2
  LC1/RConn1 -- Three-Phase Programmable Voltage Source1/RConn1
  Three-Phase Programmable Voltage Source1/LConn1 -- Ground1/LConn1
  Three-Phase Breaker/RConn1 -- LC/LConn1
  LC/LConn2 -- Three-Phase Breaker/RConn2
  Three-Phase Breaker/RConn3 -- LC/LConn3
  A/RConn1 -- Three-Phase Breaker1/LConn1 -- Three-Phase Breaker/LConn1
  B/RConn1 -- Three-Phase Breaker1/LConn2 -- Three-Phase Breaker/LConn2
  C/RConn1 -- Three-Phase Breaker1/LConn3 -- Three-Phase Breaker/LConn3
  Three-Phase Breaker1/RConn1 -- LC1/LConn1
  LC1/LConn2 -- Three-Phase Breaker1/RConn2
  Three-Phase Breaker1/RConn3 -- LC1/LConn3

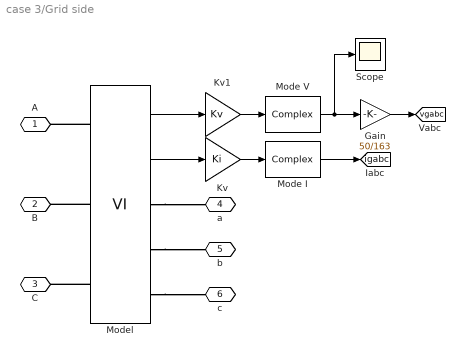
== system case 3/Grid side ==
  Gain : Gain  Gain=50/163
  Kv : Gain  Gain=Ki  SaturateOnIntegerOverflow=on  OutDataTypeStr=Inherit: Same as input  ParamDataTypeStr=Inherit: Same as input
  Kv1 : Gain  Gain=Kv  SaturateOnIntegerOverflow=on  OutDataTypeStr=Inherit: Same as input  ParamDataTypeStr=Inherit: Same as input
  Mode I : spsVIMeasurementModel/Complex
  Mode V : spsVIMeasurementModel/Complex
  Model : spsVIMeasurementModel/VI  SystemSampleTime=-1
  Scope : Scope
  A : PMIOPort  Side=Left
  B : PMIOPort  Port=2  Side=Left
  C : PMIOPort  Port=3  Side=Left
  a : PMIOPort  Port=4  Side=Right
  b : PMIOPort  Port=5  Side=Right
  c : PMIOPort  Port=6  Side=Right
  tag scope: igabc=global, vgabc=global
  wires:
  Mode I/1 -> [igabc]
  Kv1/1 -> Mode V/1
  Kv/1 -> Mode I/1
  Model/1 -> Kv1/1
  Mode V/1 -> Scope/1, Gain/1
  Model/2 -> Kv/1
  Gain/1 -> [vgabc]
  connections:
  Model/LConn1 -- A/RConn1
  Model/LConn3 -- C/RConn1
  Model/RConn3 -- c/RConn1
  Model/RConn1 -- a/RConn1
  Model/LConn2 -- B/RConn1
  Model/RConn2 -- b/RConn1

== system case 3/Results ==
  Scope : Scope  NumInputPorts=2
  Scope1 : Scope  NumInputPorts=4
  Scope2 : Scope  NumInputPorts=2
  iodmax : Constant  Value=iodmax
  iqdmax : Constant  Value=iqdmax
  wires:
  [ioq] -> Scope1/2
  [iod] -> Scope1/1
  [pdg] -> Scope2/1
  iqdmax/1 -> Scope1/4
  [qdg] -> Scope2/2
  iodmax/1 -> Scope1/3
  [vddg] -> Scope/2
  [vdgrid] -> Scope/1

== system case 3/Controller/Mean1 ==
  In : Inport  SampleTime=Ts
  Model : spsMeanValueModel/Discrete
  Subsystem : Subsystem
  Mean : Outport  SampleTime=Ts
  wires:
  In/1 -> Model/1
  Model/1 -> Subsystem/1(In1)
  Subsystem/1(Out1) -> Mean/1

== system case 3/Controller/Mean2 ==
  In : Inport  SampleTime=Ts
  Gain : Gain  Gain=3/60
  Model : spsMeanValueModel/Discrete
  Scope : Scope
  Scope1 : Scope
  Second-Order Filter : powerlib_meascontrol/Filters/Second-Order Filter  FilterType=Lowpass  Fo=10  Zeta=0.707  Ts=50e-6  Initialize=off  Vac_Init="[0,  0,  60]"  Vdc_Init=0  PlotResponse=off  FreqRange=[0, 500, 1]
      settings: SourceProductName=Simscape Power Systems  SourceProductBaseCode=PS
  Mean : Outport  SampleTime=Ts
  wires:
  In/1 -> Model/1
  Model/1 -> Scope/1, Second-Order Filter/1
  Second-Order Filter/1 -> Scope1/1, Gain/1
  Gain/1 -> Mean/1

== system case 3/Controller/NN Controller ==
  ea : Inport
  Function Fitting Neural Network : Subsystem
      mask help: Function Fitting Neural Network
      mask Display: e = 0.06;c1 = [120 150 230]/255;c2 = ([120 150 230]+0)/383;c3 = ([120 150 230]+128)/383;patch([0 1 1 0],[0 0 1 1],c1);patch([0 1 1 1-e 1-e 0+e],[0 0 1 1-e 0+e 0+e],c2);patch([0 0 1 1-e 0+e 0+e],[0 1 1 1-e 1-e 0+e],c3);plot([0 1 1 0 0],[0 0 1 1 0]);fprintf('NNET');port_label('input',1,' Input');port_label('output',1,'Output ');
  ud : Outport
  wires:
  ea/1 -> Function Fitting Neural Network/1(Input)
  Function Fitting Neural Network/1(Output) -> ud/1

== system case 3/Controller/NN Controller1 ==
  ea : Inport
  Function Fitting Neural Network : Subsystem
      mask help: Function Fitting Neural Network
      mask Display: e = 0.06;c1 = [120 150 230]/255;c2 = ([120 150 230]+0)/383;c3 = ([120 150 230]+128)/383;patch([0 1 1 0],[0 0 1 1],c1);patch([0 1 1 1-e 1-e 0+e],[0 0 1 1-e 0+e 0+e],c2);patch([0 0 1 1-e 0+e 0+e],[0 1 1 1-e 1-e 0+e],c3);plot([0 1 1 0 0],[0 0 1 1 0]);fprintf('NNET');port_label('input',1,' Input');port_label('output',1,'Output ');
  ud : Outport
  wires:
  ea/1 -> Function Fitting Neural Network/1(Input)
  Function Fitting Neural Network/1(Output) -> ud/1

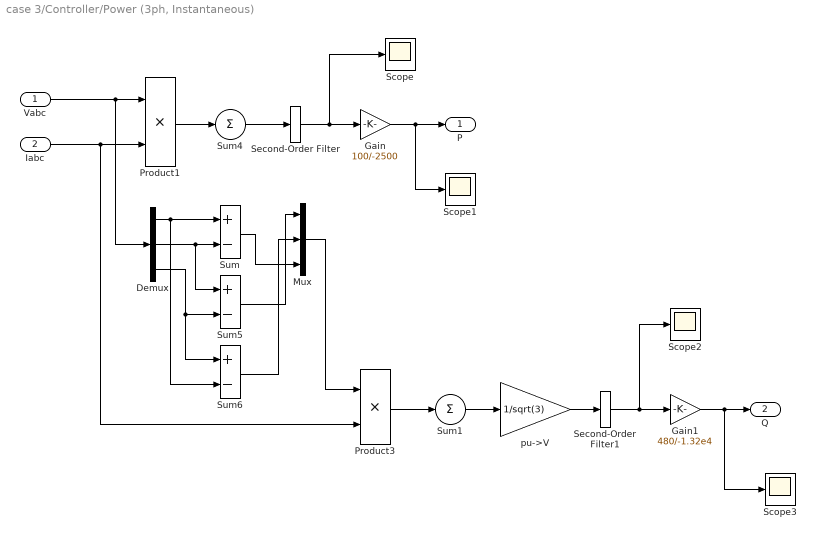
== system case 3/Controller/Power (3ph, Instantaneous) ==
  Vabc : Inport  PortDimensions=3
  Iabc : Inport  Port=2  PortDimensions=3
  Demux : Demux  Outputs=3
  Gain : Gain  Gain=100/-2500
  Gain1 : Gain  Gain=480/-1.32e4
  Mux : Mux  Inputs=3
  Product1 : Product  SaturateOnIntegerOverflow=on  InputSameDT=on  OutDataTypeStr=Inherit: Same as first input
  Product3 : Product  SaturateOnIntegerOverflow=on  InputSameDT=on  OutDataTypeStr=Inherit: Same as first input
  Scope{,1..3} (4 alike) : Scope
  Second-Order Filter : powerlib_meascontrol/Filters/Second-Order Filter  FilterType=Lowpass  Fo=10  Zeta=0.707  Ts=50e-6  Initialize=off  Vac_Init="[0,  0,  60]"  Vdc_Init=0  PlotResponse=off  FreqRange=[0, 500, 1]
      settings: SourceProductName=Simscape Power Systems  SourceProductBaseCode=PS
  Second-Order Filter1 : powerlib_meascontrol/Filters/Second-Order Filter  FilterType=Lowpass  Fo=10  Zeta=0.707  Ts=50e-6  Initialize=off  Vac_Init="[0,  0,  60]"  Vdc_Init=0  PlotResponse=off  FreqRange=[0, 500, 1]
      settings: SourceProductName=Simscape Power Systems  SourceProductBaseCode=PS
  Sum : Sum  Inputs=+-  SaturateOnIntegerOverflow=on  InputSameDT=on  OutDataTypeStr=Inherit: Same as first input
  Sum1 : Sum  Inputs=1  SaturateOnIntegerOverflow=on  InputSameDT=on  OutDataTypeStr=Inherit: Same as first input
  Sum4 : Sum  Inputs=1  SaturateOnIntegerOverflow=on  InputSameDT=on  OutDataTypeStr=Inherit: Same as first input
  Sum5 : Sum  Inputs=+-  SaturateOnIntegerOverflow=on  InputSameDT=on  OutDataTypeStr=Inherit: Same as first input
  Sum6 : Sum  Inputs=+-  SaturateOnIntegerOverflow=on  InputSameDT=on  OutDataTypeStr=Inherit: Same as first input
  pu->V : Gain  Gain=1/sqrt(3)  SaturateOnIntegerOverflow=on  OutDataTypeStr=Inherit: Same as input  ParamDataTypeStr=Inherit: Same as input
  P : Outport
  Q : Outport  Port=2
  wires:
  Product1/1 -> Sum4/1
  Vabc/1 -> Product1/1, Demux/1
  Mux/1 -> Product3/1
  Demux/2 -> Sum/2, Sum5/1
  Sum6/1 -> Mux/2
  Sum/1 -> Mux/3
  Sum4/1 -> Second-Order Filter/1
  Demux/3 -> Sum5/2, Sum6/1
  Sum5/1 -> Mux/1
  Iabc/1 -> Product1/2, Product3/2
  Product3/1 -> Sum1/1
  Sum1/1 -> pu->V/1
  Demux/1 -> Sum/1, Sum6/2
  pu->V/1 -> Second-Order Filter1/1
  Second-Order Filter1/1 -> Scope2/1, Gain1/1
  Gain/1 -> Scope1/1, P/1
  Second-Order Filter/1 -> Scope/1, Gain/1
  Gain1/1 -> Scope3/1, Q/1

== system case 3/Controller/RMS ==
  In : Inport  SampleTime=Ts
  Constant : Constant  Value=TrueRMS
  Data Type Conversion : DataTypeConversion  OutDataTypeStr=boolean
  Logical Operator : Logic  Operator=NOT  AllPortsSameDT=off  OutDataTypeStr=boolean
  "RMS " : powerlib_meascontrol/Measurements/RMS/RMS 
      settings: SourceProductName=Simscape Power Systems  SourceProductBaseCode=PS
  Subsystem : Subsystem
  Switch : Switch  Criteria=u2 ~= 0  Threshold=0.5
  "TrueRMS " : powerlib_meascontrol/Measurements/RMS/TrueRMS 
      settings: SourceProductName=Simscape Power Systems  SourceProductBaseCode=PS
  RMS : Outport  SampleTime=Ts
  wires:
  "RMS "/1 -> Switch/3
  "TrueRMS "/1 -> Switch/1
  Logical Operator/1 -> "RMS "/Enable
  Data Type Conversion/1 -> Logical Operator/1, "TrueRMS "/Enable, Switch/2
  In/1 -> "TrueRMS "/1, "RMS "/1
  Constant/1 -> Data Type Conversion/1
  Switch/1 -> Subsystem/1(In1)
  Subsystem/1(Out1) -> RMS/1

== system case 3/Controller/RMS4 ==
  In : Inport  SampleTime=Ts
  Constant : Constant  Value=TrueRMS
  Data Type Conversion : DataTypeConversion  OutDataTypeStr=boolean
  Logical Operator : Logic  Operator=NOT  AllPortsSameDT=off  OutDataTypeStr=boolean
  Mean1 : Subsystem  DialogController=POWERSYS.PowerSysDialog  LoadFcn=sps_rtmsupport('LoadFcn', gcbh);  StartFcn=sps_rtmsupport('StartFcn', gcbh);  StopFcn=sps_rtmsupport('StopFcn', gcbh);  mask(Mean){Freq=50, Vinit=0, Ts=50e-6}
      mask prompts: Freq "Fundamental frequency (Hz):"; Vinit "Initial input (DC component):"; Ts "Sample time:"
      mask help: Compute the mean value of the input signal over a running window of one cycle of the specified fundamental frequency. For the first cycle of simulation, the output is held constant to the specified initial input value.
      mask init:
      | block=gcb;
      | [WantBlockChoice,Ts,sps] = powericon('MeanInit',block,Freq,Vinit,Ts);
      | powericon('SetInternalModels','set',block,WantBlockChoice);
      settings: CopyFcn=sps_rtmsupport('CopyFcn', gcbh);  DeleteFcn=sps_rtmsupport('DeleteFcn', gcbh);  UndoDeleteFcn=sps_rtmsupport('UndoDeleteFcn', gcbh);  ModelCloseFcn=sps_rtmsupport('ModelCloseFcn', gcbh);  PreSaveFcn=sps_rtmsupport('PreSaveFcn', gcbh);  PostSaveFcn=sps_rtmsupport('PostSaveFcn', gcbh);  NameChangeFcn=sps_rtmsupport('NameChangeFcn', gcbh);  PreCopyFcn=sps_rtmsupport('PreCopyFcn', gcbh);  OpenFcn=sps_rtmsupport('OpenFcn', gcbh, []);  CloseFcn=sps_rtmsupport('CloseFcn', gcbh);  PreDeleteFcn=sps_rtmsupport('PreDeleteFcn', gcbh);
      mask Help: helpview(psbhelp);
      mask Display:
      | plot(0,0, 1,1)
      | plot([0.8 1], [0.75 0.75])
      | plot([0.85 .95], [0.35 0.65],[0.85 .95], [0.65 0.35])
  "RMS " : powerlib_meascontrol/Measurements/RMS/RMS 
      settings: SourceProductName=Simscape Power Systems  SourceProductBaseCode=PS
  Scope : Scope
  Subsystem : Subsystem
  Switch : Switch  Criteria=u2 ~= 0  Threshold=0.5
  "TrueRMS " : powerlib_meascontrol/Measurements/RMS/TrueRMS 
      settings: SourceProductName=Simscape Power Systems  SourceProductBaseCode=PS
  RMS : Outport  SampleTime=Ts
  wires:
  Subsystem/1(RMS) -> RMS/1
  Constant/1 -> Data Type Conversion/1
  Logical Operator/1 -> "RMS "/Enable
  Data Type Conversion/1 -> Switch/2, "TrueRMS "/Enable, Logical Operator/1
  Switch/1 -> Subsystem/1(In2), Scope/1
  In/1 -> "RMS "/1, "TrueRMS "/1
  "RMS "/1 -> Switch/3
  "TrueRMS "/1 -> Switch/1

== system case 3/Controller/abc-abc ==
  In1 : Inport
  Selector : Selector  InputPortWidth=3  IndexOptions=Index vector (dialog)  Indices=[1]  OutputSizes=1
  abc to dq5 : powerlib_meascontrol/Transformations/abc to dq0  Alignment=90 degrees behind phase A axis
  dq0 to abc1 : powerlib_meascontrol/Transformations/dq0 to abc  Alignment=90 degrees behind phase A axis
  Out1 : Outport
  tag scope: vdgrid=global
  wires:
  [rowg] -> abc to dq5/2, dq0 to abc1/2
  In1/1 -> abc to dq5/1
  abc to dq5/1 -> Selector/1, dq0 to abc1/1
  dq0 to abc1/1 -> Out1/1
  Selector/1 -> [vdgrid]

== system case 3/Controller/abc-abc1 ==
  In1 : Inport
  Selector : Selector  InputPortWidth=3  IndexOptions=Index vector (dialog)  Indices=[1]  OutputSizes=1
  abc to dq5 : powerlib_meascontrol/Transformations/abc to dq0  Alignment=90 degrees behind phase A axis
  dq0 to abc1 : powerlib_meascontrol/Transformations/dq0 to abc  Alignment=90 degrees behind phase A axis
  Out1 : Outport
  tag scope: vddg=global
  wires:
  Selector/1 -> [vddg]
  dq0 to abc1/1 -> Out1/1
  abc to dq5/1 -> dq0 to abc1/1, Selector/1
  In1/1 -> abc to dq5/1
  [rowdg] -> dq0 to abc1/2, abc to dq5/2

== system case 3/DG side/Subsystem ==
  In1 : Inport
  Gain1 : Gain  Gain=1/100
  Multiply5 : Product
  RMS : powerlib_meascontrol/Measurements/RMS  TrueRMS=on  Freq=50  RMSInit=120  Ts=50e-6
  Scope : Scope
  Out2 : Outport
  wires:
  [vgabc] -> Multiply5/2
  Gain1/1 -> Multiply5/1
  RMS/1 -> Gain1/1
  In1/1 -> RMS/1
  Multiply5/1 -> Out2/1, Scope/1

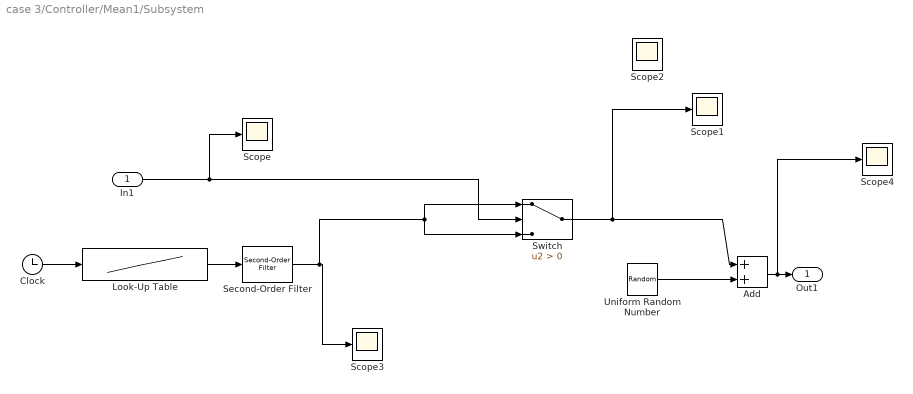
== system case 3/Controller/Mean1/Subsystem ==
  In1 : Inport
  Add : Sum
  Clock : Clock
  Look-Up Table : Lookup  InputValues=[0 2 2.01 6]  Table=[-0.01 -0.01 -12 -12]  SaturateOnIntegerOverflow=on
  Scope{,1..4} (5 alike) : Scope
  Second-Order Filter : powerlib_meascontrol/Filters/Second-Order Filter  FilterType=Lowpass  Fo=10  Zeta=0.909  Ts=50e-6  Initialize=off  Vac_Init="[0,  0,  60]"  Vdc_Init=0  PlotResponse=off  FreqRange=[0, 500, 1]
      settings: SourceProductName=Simscape Power Systems  SourceProductBaseCode=PS
  Switch : Switch  Criteria=u2 > Threshold
  Uniform Random Number : UniformRandomNumber  Minimum=-0.1  Maximum=0.1  SampleTime=50e-6
  Out1 : Outport
  wires:
  Clock/1 -> Look-Up Table/1
  Look-Up Table/1 -> Second-Order Filter/1
  In1/1 -> Switch/2, Scope/1
  Second-Order Filter/1 -> Switch/1, Switch/3, Scope3/1
  Switch/1 -> Add/1, Scope1/1
  Add/1 -> Scope4/1, Out1/1
  Uniform Random Number/1 -> Add/2

== system case 3/Controller/NN Controller/Function Fitting Neural Network ==
  Input : Inport  PortDimensions=1
      mask Display: e = 0.06;c1 = [120 230 180]/255;c2 = ([120 230 180]+0)/(256+128);c3 = ([120 230 180]+128)/(256+128);patch([0 1 1 0],[0 0 1 1],c1);patch([0 1 1 1-e 1-e 0+e],[0 0 1 1-e 0+e 0+e],c2);patch([0 0 1 1-e 0+e 0+e],[0 1 1 1-e 1-e 0+e],c3);plot([0 1 1 0 0],[0 0 1 1 0]);
  Layer 1 : Subsystem
      mask Display: e = 0.06;c1 = [120 150 230]/255;c2 = ([120 150 230]+0)/383;c3 = ([120 150 230]+128)/383;patch([0 1 1 0],[0 0 1 1],c1);patch([0 1 1 1-e 1-e 0+e],[0 0 1 1-e 0+e 0+e],c2);patch([0 0 1 1-e 0+e 0+e],[0 1 1 1-e 1-e 0+e],c3);plot([0 1 1 0 0],[0 0 1 1 0]);
  Layer 2 : Subsystem
      mask Display: e = 0.06;c1 = [120 150 230]/255;c2 = ([120 150 230]+0)/383;c3 = ([120 150 230]+128)/383;patch([0 1 1 0],[0 0 1 1],c1);patch([0 1 1 1-e 1-e 0+e],[0 0 1 1-e 0+e 0+e],c2);patch([0 0 1 1-e 0+e 0+e],[0 1 1 1-e 1-e 0+e],c3);plot([0 1 1 0 0],[0 0 1 1 0]);
  Process Input 1 : Subsystem
      mask Display: e = 0.06;c1 = [120 150 230]/255;c2 = ([120 150 230]+0)/383;c3 = ([120 150 230]+128)/383;patch([0 1 1 0],[0 0 1 1],c1);patch([0 1 1 1-e 1-e 0+e],[0 0 1 1-e 0+e 0+e],c2);patch([0 0 1 1-e 0+e 0+e],[0 1 1 1-e 1-e 0+e],c3);plot([0 1 1 0 0],[0 0 1 1 0]);
  Process Output 1 : Subsystem
      mask Display: e = 0.06;c1 = [120 150 230]/255;c2 = ([120 150 230]+0)/383;c3 = ([120 150 230]+128)/383;patch([0 1 1 0],[0 0 1 1],c1);patch([0 1 1 1-e 1-e 0+e],[0 0 1 1-e 0+e 0+e],c2);patch([0 0 1 1-e 0+e 0+e],[0 1 1 1-e 1-e 0+e],c3);plot([0 1 1 0 0],[0 0 1 1 0]);
  Output : Outport  InitialOutput=0
      mask Display: e = 0.06;c1 = [120 230 180]/255;c2 = ([120 230 180]+0)/(256+128);c3 = ([120 230 180]+128)/(256+128);patch([0 1 1 0],[0 0 1 1],c1);patch([0 1 1 1-e 1-e 0+e],[0 0 1 1-e 0+e 0+e],c2);patch([0 0 1 1-e 0+e 0+e],[0 1 1 1-e 1-e 0+e],c3);plot([0 1 1 0 0],[0 0 1 1 0]);
  wires:
  Input/1 -> Process Input 1/1(x)
  Process Output 1/1(y) -> Output/1
  Process Input 1/1(p) -> Layer 1/1("p{1}")
  Layer 1/1("a{1}") -> [feedback1]
  [feedback1] -> Layer 2/1("a{1} ")
  Layer 2/1("a{2}") -> Process Output 1/1(a)
